simulink model "Unicorn_Demo2"  (R2015a)
settings: Solver=FixedStepDiscrete  StartTime=0.0  StopTime=inf  RelTol=1e-3
undefined symbols (not defined in the file): fdesignblkfcn, gcbh, UN
libraries: dsparch4 x3, UnicornLib x1
settings Model: Creator=reitner  LastModifiedBy=walchshofer
settings DebuggingCC: FrameProcessingCompatibilityMsg=none

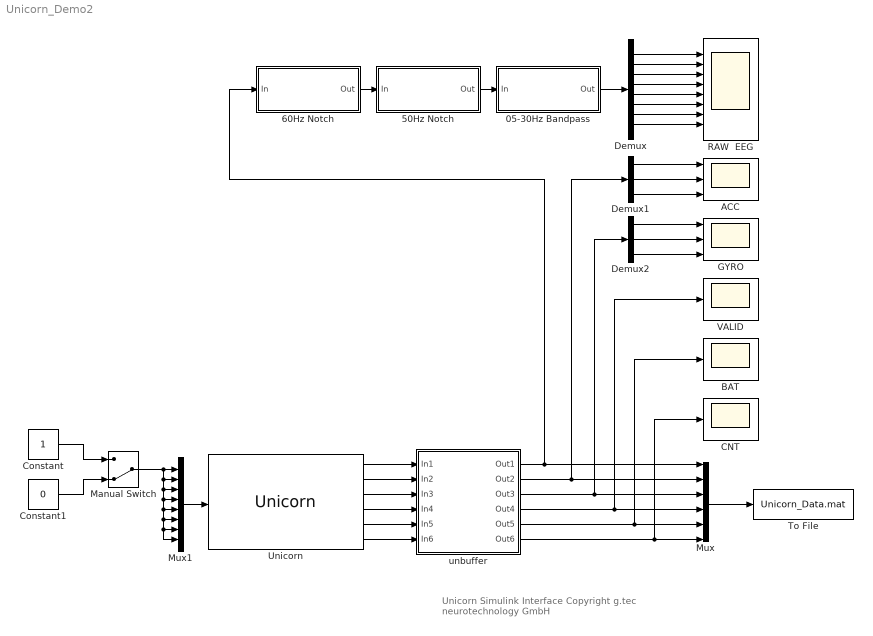
== system Unicorn_Demo2 ==
  note: Unicorn Simulink Interface
      | Copyright g.tec neurotechnology GmbH
  05-30Hz Bandpass : Subsystem  DialogController=fdesignblkfcn  InitFcn=fdesignblkfcn(gcbh, {'InitFcn'});  mask(Bandpass Filter){}
      mask help: Design a bandpass filter
      settings: CopyFcn=fdesignblkfcn(gcbh, {'CopyFcn'});
      mask Help: helpview(mapfilelocation('dsp'), 'dspbandpassfilter');
      mask Display: disp('Bandpass');
  50Hz Notch : Subsystem  DialogController=fdesignblkfcn  InitFcn=fdesignblkfcn(gcbh, {'InitFcn'});  mask(Bandstop Filter){}
      mask help: Design a bandstop filter
      settings: CopyFcn=fdesignblkfcn(gcbh, {'CopyFcn'});
      mask Help: helpview(mapfilelocation('dsp'), 'dspbandstopfilter');
      mask Display: disp('Bandstop');
  60Hz Notch : Subsystem  DialogController=fdesignblkfcn  InitFcn=fdesignblkfcn(gcbh, {'InitFcn'});  mask(Bandstop Filter){}
      mask help: Design a bandstop filter
      settings: CopyFcn=fdesignblkfcn(gcbh, {'CopyFcn'});
      mask Help: helpview(mapfilelocation('dsp'), 'dspbandstopfilter');
      mask Display: disp('Bandstop');
  "ACC " : Scope  NumInputPorts=3
      settings: YMin=-10~-10~-10  YMax=10~10~10  MaxDataPoints=2500
  BAT : Scope
      settings: YMin=0  YMax=100  SaveName=ScopeData4  MaxDataPoints=2500
  CNT : Scope
      settings: YMin=0  YMax=2500  SaveName=ScopeData5  MaxDataPoints=2500
  Constant : Constant  OutDataTypeStr=boolean
  Constant1 : Constant  Value=0  OutDataTypeStr=boolean
  Demux : Demux  Outputs=8
  Demux1 : Demux  Outputs=3
  Demux2 : Demux  Outputs=3
  GYRO : Scope  NumInputPorts=3
      settings: YMin=-1000~-1000~-1000  YMax=1000~1000~1000  SaveName=ScopeData2  MaxDataPoints=2500
  Manual Switch : ManualSwitch  CurrentSetting=0
  Mux : Mux  Inputs=6
  Mux1 : Mux  Inputs=8
  RAW  EEG : Scope  NumInputPorts=8
      settings: TickLabels=off  YMin=-350~-450~10~-50~-140~325~-100~-475  YMax=-175~-200~150~80~0~500~20~-300  MaxDataPoints=2500
  To File : ToFile  Filename=Unicorn_Data.mat  MatrixName=y
  Unicorn : UnicornLib/Unicorn  serial=UN-2016.01.01  old_serial=UN-2016.01.01  frame_length=1  input_source=Electrode
  VALID : Scope
      settings: YMin=0  YMax=1  SaveName=ScopeData3  MaxDataPoints=2500
  "unbuffer " : Subsystem
      mask Display:
      | port_label('input',1,'EEG')
      | port_label('input',2,'ACC')
      | port_label('input',3,'GYRO')
      | port_label('input',4,'VALID')
      | port_label('input',5,'BAT')
      | port_label('input',6,'CNT')
      | port_label('output',1,'EEG')
      | port_label('output',2,'ACC')
      | port_label('output',3,'GYRO')
      | port_label('output',4,'VALID')
      | port_label('output',5,'BAT')
      | port_label('output',6,'CNT')
  wires:
  Demux/8 -> RAW  EEG/8
  Demux/7 -> RAW  EEG/7
  Demux/6 -> RAW  EEG/6
  Demux/5 -> RAW  EEG/5
  Demux/4 -> RAW  EEG/4
  Demux/3 -> RAW  EEG/3
  Demux/2 -> RAW  EEG/2
  Demux/1 -> RAW  EEG/1
  Demux1/1 -> "ACC "/1
  Demux1/2 -> "ACC "/2
  Demux1/3 -> "ACC "/3
  Demux2/1 -> GYRO/1
  Demux2/2 -> GYRO/2
  Demux2/3 -> GYRO/3
  "unbuffer "/1(Out1) -> 60Hz Notch/1(In), Mux/1
  "unbuffer "/2(Out2) -> Mux/2, Demux1/1
  "unbuffer "/3(Out3) -> Mux/3, Demux2/1
  "unbuffer "/4(Out4) -> Mux/4, VALID/1
  "unbuffer "/5(Out5) -> Mux/5, BAT/1
  "unbuffer "/6(Out6) -> Mux/6, CNT/1
  Unicorn/1 -> "unbuffer "/1(In1)
  Unicorn/2 -> "unbuffer "/2(In2)
  Unicorn/3 -> "unbuffer "/3(In3)
  Unicorn/4 -> "unbuffer "/4(In4)
  Unicorn/5 -> "unbuffer "/5(In5)
  Unicorn/6 -> "unbuffer "/6(In6)
  Mux/1 -> To File/1
  Constant/1 -> Manual Switch/1
  Constant1/1 -> Manual Switch/2
  Mux1/1 -> Unicorn/1
  Manual Switch/1 -> Mux1/8, Mux1/7, Mux1/6, Mux1/5, Mux1/4, Mux1/3, Mux1/2, Mux1/1
  60Hz Notch/1(Out) -> 50Hz Notch/1(In)
  50Hz Notch/1(Out) -> 05-30Hz Bandpass/1(In)
  05-30Hz Bandpass/1(Out) -> Demux/1

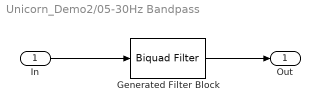
== system Unicorn_Demo2/05-30Hz Bandpass ==
  In : Inport
  Generated Filter Block : dsparch4/Biquad Filter  Tag=BlockMethodSubSystem  IIRFiltStruct=Direct form II  CoeffSource=Specify via dialog  BiQuadCoeffs=[0.4322526152450743 0 -0.4322526152450743 1 -1.0011806751735479 0.3599418394747359;0.089147308745349971 0 -0.089147308745349971 1 -0.90316691443797437 0.21573805671244461;0.0088211325061849071 0 -0.0088211325061849071 1 -1.9935355151831708 0.99369356215971294;0.012337659349727709 0 -0.012337659349727709 1 -1.9822422643876501 0.98240374527709184;2 0 -2 1 -1.9751756853515128 0.97534142261558909;2 0 -2 1 -1.2458737431168365 0.70689135033598349]  a0Flag=Warning  IC=0  ICnum=0  ICden=0  denAccumFracLength=30  denProdOutputFracLength=30  secondMemoryFracLength=15  roundingMode=Floor  overflowMode=off  ScaleValues=[0.35278894395693888;1;1;1;1;1;133.18750137787509]  optimizeScaleValues=on  ScaleValueMode=Specify via input port (g)  scaleValueFracLength=14  FilterSource=Specify via dialog  FilterObject=Hm_biquad
  Out : Outport
  wires:
  In/1 -> Generated Filter Block/1
  Generated Filter Block/1 -> Out/1

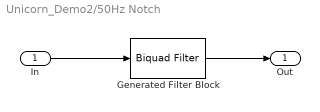
== system Unicorn_Demo2/50Hz Notch ==
  In : Inport
  Generated Filter Block : dsparch4/Biquad Filter  Tag=BlockMethodSubSystem  IIRFiltStruct=Direct form II  CoeffSource=Specify via dialog  BiQuadCoeffs=[2 -1.2376311593598059 1.9999999999999996 1 -0.58917542534408363 0.90420359373902093]  a0Flag=Warning  IC=0  ICnum=0  ICden=0  denAccumFracLength=30  denProdOutputFracLength=30  secondMemoryFracLength=15  roundingMode=Floor  overflowMode=off  ScaleValues=[0.091083863875771748;5.226511899890804]  optimizeScaleValues=on  ScaleValueMode=Specify via input port (g)  scaleValueFracLength=14  FilterSource=Specify via dialog  FilterObject=Hm_biquad
  Out : Outport
  wires:
  Generated Filter Block/1 -> Out/1
  In/1 -> Generated Filter Block/1

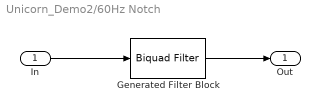
== system Unicorn_Demo2/60Hz Notch ==
  In : Inport
  Generated Filter Block : dsparch4/Biquad Filter  Tag=BlockMethodSubSystem  IIRFiltStruct=Direct form II  CoeffSource=Specify via dialog  BiQuadCoeffs=[1.9999999999999998 -0.25147970790103907 2 1 -0.11971714088439944 0.90420359373902071]  a0Flag=Warning  IC=0  ICnum=0  ICden=0  denAccumFracLength=30  denProdOutputFracLength=30  secondMemoryFracLength=15  roundingMode=Floor  overflowMode=off  ScaleValues=[0.095607010933771011;4.9792467496397919]  optimizeScaleValues=on  ScaleValueMode=Specify via input port (g)  scaleValueFracLength=14  FilterSource=Specify via dialog  FilterObject=Hm_biquad
  Out : Outport
  wires:
  Generated Filter Block/1 -> Out/1
  In/1 -> Generated Filter Block/1

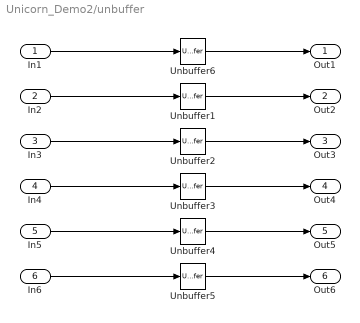
== system Unicorn_Demo2/unbuffer  ==
  In1 : Inport
  In2 : Inport  Port=2
  In3 : Inport  Port=3
  In4 : Inport  Port=4
  In5 : Inport  Port=5
  In6 : Inport  Port=6
  Unbuffer{1..6} (6 alike) : Unbuffer
  Out1 : Outport
  Out2 : Outport  Port=2
  Out3 : Outport  Port=3
  Out4 : Outport  Port=4
  Out5 : Outport  Port=5
  Out6 : Outport  Port=6
  wires:
  In1/1 -> Unbuffer6/1
  In6/1 -> Unbuffer5/1
  In2/1 -> Unbuffer1/1
  In3/1 -> Unbuffer2/1
  In4/1 -> Unbuffer3/1
  In5/1 -> Unbuffer4/1
  Unbuffer4/1 -> Out5/1
  Unbuffer5/1 -> Out6/1
  Unbuffer3/1 -> Out4/1
  Unbuffer2/1 -> Out3/1
  Unbuffer1/1 -> Out2/1
  Unbuffer6/1 -> Out1/1
